simulink model "Simple_Model_Packaging_5_1"  (R2022b)
settings: Solver=VariableStepAuto  StartTime=0.0  StopTime=0.01  RelTol=1e-3
PreLoadFcn:
  | Parameter_Initialize_5
InitFcn:
  | Parameter_Initialize_5
undefined symbols (not defined in the file or in its folder): gcbh, magnitude, model, rcfiltgaincompat
libraries: commfilt2 x1, simulink x1
settings Model: Creator=z0y  LastModifiedBy=z0y

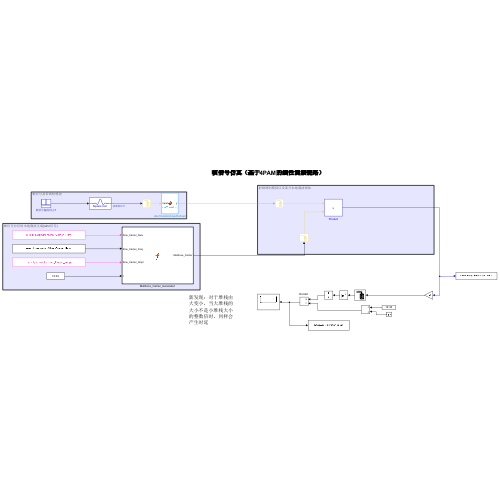
[thumbnail: Simulink's stored preview of the top-level diagram]
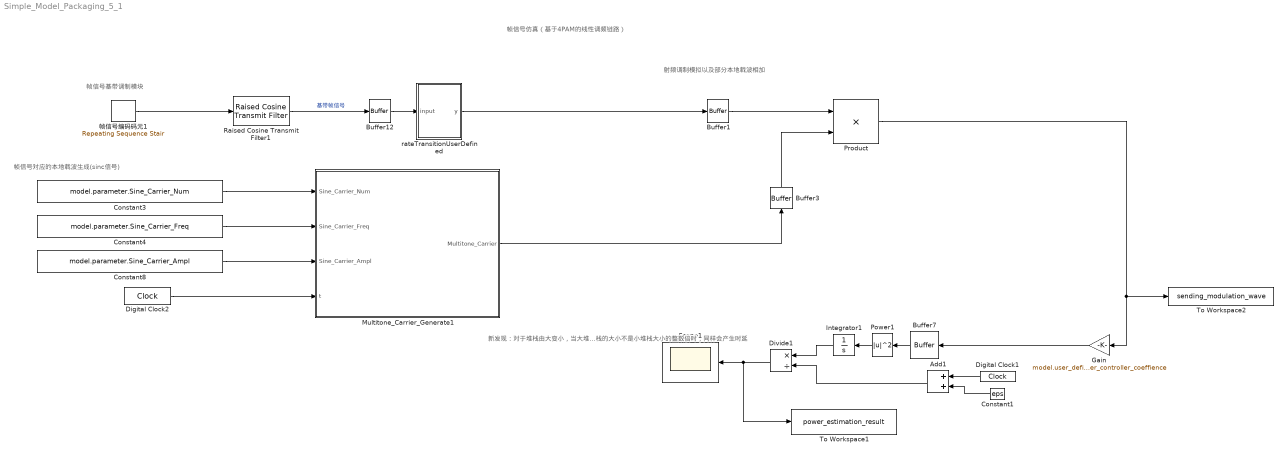
== system Simple_Model_Packaging_5_1 ==
  note: 新发现：对于堆栈由大变小，当大堆栈的大小不是小堆栈大小的整数倍时，同样会产生时延
  note: 射频调制模拟以及部分本地载波相加
  note: 帧信号仿真（基于4PAM的线性调频链路）
  note: 帧信号对应的本地载波生成(sinc信号)
  note: 帧信号基带调制模块
  Add1 : Sum
  Buffer1 : Buffer  N=model.parameter.Raised_Cosine_Transmit_Filter.Output_samples_per_symbol  OutputFrames=off
  Buffer12 : Buffer  N=model.parameter.Buffer12.Output_buffer_size  OutputFrames=off
  Buffer3 : Buffer  N=model.parameter.Raised_Cosine_Transmit_Filter.Output_samples_per_symbol  OutputFrames=off
  Buffer7 : Buffer  N=1  OutputFrames=off
  Constant1 : Constant  Value=eps  SampleTime=model.parameter.channel_estimate_fs
  Constant3 : Constant  Value=model.parameter.Sine_Carrier_Num
  Constant4 : Constant  Value=model.parameter.Sine_Carrier_Freq
  Constant8 : Constant  Value=model.parameter.Sine_Carrier_Ampl
  Digital Clock1 : DigitalClock  SampleTime=model.parameter.channel_estimate_fs
  Digital Clock2 : DigitalClock  SampleTime=model.parameter.Digital_Clock2.CarrierTs
  Divide1 : Product  Inputs=*/
  Gain : Gain  Gain=model.user_defined.TR.Sig_power_controller_coeffience
  Integrator1 : Integrator
  Multitone_Carrier_Generate1 : MATLAB Function  TreatAsAtomicUnit=on
  Power1 : Math  Operator=magnitude^2
  Product : Product
  Raised Cosine Transmit Filter1 : commfilt2/Raised Cosine Transmit Filter  filtType=Square root  R=model.parameter.Raised_Cosine_Transmit_Filter.Rolloff_factor  filtSpan=model.parameter.Raised_Cosine_Transmit_Filter.Filter_span_in_symbols  N=model.parameter.Raised_Cosine_Transmit_Filter.Output_samples_per_symbol  filterGain=rcfiltgaincompat(gcbh)  InputProcessing=Columns as channels (frame based)  RateOptions=Enforce single-rate processing  framing=Mute  checkCoeff=off  variableName=rcTxFilt1  checkGain=Normalized  sampMode=Mute  saveAsFlag=0  currentFiltSpan=10  D=(10)/2  launchFVT=on  roundingMode=Floor  overflowMode=off  coeffDataTypeStr=Inherit: Same word length as input  coeffMin=[]  coeffMax=[]  coeffLastDataTypeStr=Inherit: Same word length as input  outputDataTypeStr=Inherit: Same as accumulator  outputMin=[]  outputMax=[]  outputLastDataTypeStr=Inherit: Same as accumulator
  Scope1 : Scope
  To Workspace1 : ToWorkspace  VariableName=power_estimation_result  SaveFormat=Timeseries  SampleTime=-1
  To Workspace2 : ToWorkspace  VariableName=sending_modulation_wave  SaveFormat=Timeseries  SampleTime=-1
  rateTransitionUserDefined : MATLAB Function  TreatAsAtomicUnit=on
  帧信号编码码元1 : simulink/Sources/Repeating Sequence Stair  OutValues=model.parameter.Repeating_Sequence_Stair.output_vector  tsamp=model.parameter.Repeating_Sequence_Stair.CodeTs  OutMin=[]  OutMax=[]  OutDataTypeStr=double  OutputDataTypeScalingMode=double  OutDataType=fixdt(0,8)  ConRadixGroup=Best Precision: Vector-wise  OutScaling=2^-12
  wires:
  Power1/1 -> Integrator1/1
  Buffer3/1 -> Product/2
  Gain/1 -> Buffer7/1
  Digital Clock1/1 -> Add1/1
  Buffer7/1 -> Power1/1
  Buffer1/1 -> Product/1
  Constant1/1 -> Add1/2
  Product/1 -> To Workspace2/1, Gain/1
  Integrator1/1 -> Divide1/1
  Add1/1 -> Divide1/2
  Divide1/1 -> To Workspace1/1, Scope1/1
  帧信号编码码元1/1 -> Raised Cosine Transmit Filter1/1
  Constant4/1 -> Multitone_Carrier_Generate1/2(Sine_Carrier_Freq)
  Digital Clock2/1 -> Multitone_Carrier_Generate1/4(t)
  Constant8/1 -> Multitone_Carrier_Generate1/3(Sine_Carrier_Ampl)
  Constant3/1 -> Multitone_Carrier_Generate1/1(Sine_Carrier_Num)
  Buffer12/1 -> rateTransitionUserDefined/1(input)
  rateTransitionUserDefined/1(y) -> Buffer1/1
  Raised Cosine Transmit Filter1/1 -> Buffer12/1  "基带帧信号"
  Multitone_Carrier_Generate1/1(Multitone_Carrier) -> Buffer3/1

== matlab function Simple_Model_Packaging_5_1/Multitone_Carrier_Generate1 ==
  data: Sine_Carrier_Num input; Multitone_Carrier output; Sine_Carrier_Freq input; Sine_Carrier_Ampl input; t input
function Multitone_Carrier = fcn(Sine_Carrier_Num, Sine_Carrier_Freq, Sine_Carrier_Ampl, t)
    Multitone_Carrier = complex(0);
    for index = 1:Sine_Carrier_Num
            Multitone_subCarrier = Sine_Carrier_Ampl(index) * exp(1j*2*pi*Sine_Carrier_Freq(index)*t);
            Multitone_Carrier = Multitone_Carrier + Multitone_subCarrier;
    end
end

== matlab function Simple_Model_Packaging_5_1/rateTransitionUserDefined ==
  data: y output; input input
% function y = carrierGenerator(t)
%     fc = 5e6;
%     y = exp(1i*2*pi*fc*t);

function y = rateTransition(input)
%     global rateFactor;
%     p = rateFactor;
    p = 10;
    q = 1;
    y = resample(input,p,q);
%     y(1:100) = repmat(y(100),1,100);
%     y(end-99:end) = repmat(y(end-99),1,100);
end
